simulink model "PMSM_Simulation"  (R2023a)
settings: Solver=ode23t  StartTime=0.0  StopTime=5  MaxStep=0.2  RelTol=1e-4  EnableMultiTasking=on
InitFcn:
  | p = 4;
  | Ld = 0.000425;
  | Lq = 0.00085;
  | psim = 0.119489;
  | Rs = 0.0485;
  | J = 0.00027;
  | Kpwm = 1;
  | Tsi = 0.0001;
  | h = 900;
  | 
  | L0 = (Ld+Lq)/2;
  | SMO_Kp = 100;
  | SMO_Coef =0.0001;
  | Ki_id = Ld*(h+1)/(4.5*Kpwm*(Tsi^2)*(h^2));
  | Kp_id = Ld*(h+1)/(4.5*Kpwm*Tsi*h);
  | 
  | wc =3000;
  | 
  | Ki_iq = Lq*(h+1)/(4.5*Kpwm*Tsi^2*h^2);
  | Kp_iq = Lq*(h+1)/(4.5*Kpwm*Tsi*h);
  | 
  | 
  | Kp_Spd = pi*J/(300*p*psim*Tsi)
  | Ki_Spd = pi*J/(6000*p*psim*Tsi^2)
  | 
  | DeadTime = 2e-6;
  | 
  | Udc = 650;
model workspace (MAT data in the model file):
  KfDeadCompen_CpPeriodTimesT_NULL = Simulink.Parameter
  KfDeadCompen_CpPeriodTimesT_NULL.Value = 0
  KfDeadCompen_CpPeriodTimesT_NULL.DataType = 'single'
  KfDeadCompen_CpPeriodTimesT_NULL.Complexity = 'real'
  KfDeadCompen_CpPeriodTimesT_NULL.Dimensions = [1 1]
  KfMDCC_InvParkCpPeriodTimesT_NULL = Simulink.Parameter
  KfMDCC_InvParkCpPeriodTimesT_NULL.Value = 0
  KfMDCC_InvParkCpPeriodTimesT_NULL.DataType = 'single'
  KfMDCC_InvParkCpPeriodTimesT_NULL.Complexity = 'real'
  KfMDCC_InvParkCpPeriodTimesT_NULL.Dimensions = [1 1]
values from neighbouring files (symbols this model uses):
  KfDeadCompen_SetDeltaTime_us = myPackage.Parameter    [DeadCompen.m]
  VbDeadComp_SwtUseIsttrDes_flg = myPackage.Parameter    [DeadCompen.m]
  VfDeadCompen_agIPredAdpr_C = myPackage.Parameter    [DeadCompen.m]
  VfDeadCompen_ISttrDdeThdSwt_A = myPackage.Parameter    [DeadCompen.m]
  VfDeadCompen_ISttrIgbtThdSwt_A = myPackage.Parameter    [DeadCompen.m]
  VfDeadCompen_rDdeISttrHi_R = myPackage.Parameter    [DeadCompen.m]
  VfDeadCompen_rDdeISttrLo_R = myPackage.Parameter    [DeadCompen.m]
  VfDeadCompen_rIgbtISttrHi_R = myPackage.Parameter    [DeadCompen.m]
  VfDeadCompen_rIgbtISttrLo_R = myPackage.Parameter    [DeadCompen.m]
  VfDeadCompen_uDdeISttrHi_V = myPackage.Parameter    [DeadCompen.m]
  VfDeadCompen_uDdeISttrLo_V = myPackage.Parameter    [DeadCompen.m]
  VfDeadCompen_uIgbtISttrHi_V = myPackage.Parameter    [DeadCompen.m]
  VfDeadCompen_uIgbtISttrLo_V = myPackage.Parameter    [DeadCompen.m]
undefined symbols (not defined in the file or in its folder): DiscIntNeverNeededParam, TableDeadTime_us, TableDeadTimeLookUpCur_A, VuDeadCompen_agIPredAdpr_C
libraries: simulink x23, mcbcontrolslib x11, mcbplantlib x1, spsCurrentMeasurementLib x1, spsDCVoltageSourceLib x1, spsMultimeterLib x1, spsPermanentMagnetSynchronousMachineLib x1, eePmsmCurrentController x1, spsThreePhaseVIMeasurementLib x1, spsUniversalBridgeLib x1, spspowerguiLib x1
(part 1 of 4)
settings Model: SimulationMode=accelerator  Creator=洲  LastModifiedBy=洲
settings SolverCC: AlgebraicLoopSolver=TrustRegion  MaxZcPerStep=1
settings DataIOCC: LimitDataPoints=on  MaxDataPoints=10000
settings OptimizationCC: ReuseModelBlockBuffer=off  LifeSpan=inf
settings DebuggingCC: AllowSymbolicDim=off  SFUnexpectedBacktrackingDiag=warning  SFNoUnconditionalDefaultTransitionDiag=warning  SFExecutionAtInitializationDiag=none  ArithmeticOperatorsInVariantConditions=warning
settings ModelReferenceCC: EnableRefExpFcnMdlSchedulingChecks=on
settings SFSimCC: SimUseLocalCustomCode=off  CustomCodeUndefinedFunction=UseInterfaceOnly
settings RTWCC: RTWUseLocalCustomCode=off  DLArmComputeVersion=19.05
settings CodeAppCC: StateflowObjectComments=on
settings GRTTargetCC: TargetLangStandard=C89/C90 (ANSI)
settings ConfigComp: CovMetricSettings=dw  CovSaveCumulativeToWorkspaceVar=on  CovSaveSingleToWorkspaceVar=on  CovExternalEMLEnable=off  CovSFcnEnable=off
settings SimscapeCC: SimscapeLogType=all  SimscapeLogDataHistory=10000

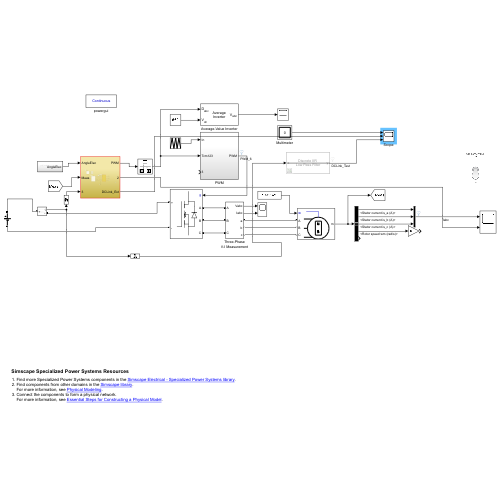
[thumbnail: Simulink's stored preview of the top-level diagram]
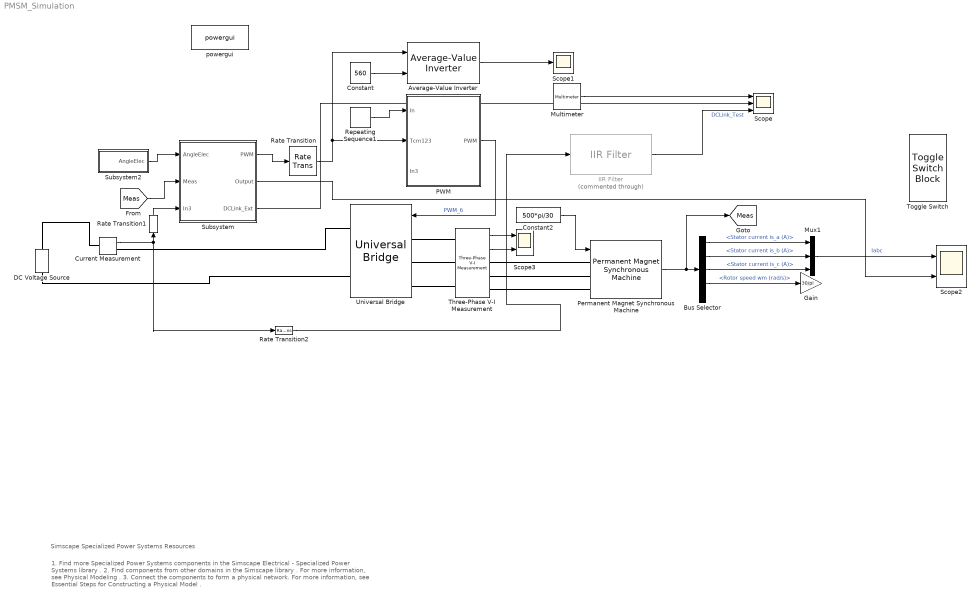
== system PMSM_Simulation ==
  note: 1. Find more Specialized Power Systems components in the Simscape Electrical - Specialized Power Systems library .
      | 2. Find components from other domains in the Simscape library .
      | For more information, see Physical Modeling .
      | 3. Connect the components to form a physical network.
      | For more information, see Essential Steps for Constructing a Physical Model .
  note: Simscape Specialized Power Systems Resources
  Average-Value Inverter : mcbplantlib/Average-Value Inverter
      settings: LibrarySourceBlock=mcblib/Electrical Systems/Inverters/Average-Value Inverter
  Bus Selector : BusSelector  OutputSignals=Stator current is_a (A),Stator current is_b (A),Stator current is_c (A),Rotor speed wm (rad/s),Electromagnetic torque Te (N*m)
  Constant : Constant  Value=560
  Constant2 : Constant  Value=500*pi/30
  Current Measurement : spsCurrentMeasurementLib/Current Measurement  PhasorSimulation=off  OutputType=Complex  PSBequivalent=0
  DC Voltage Source : spsDCVoltageSourceLib/DC Voltage Source  Amplitude=650  Measurements=None
  Gain : Gain  Gain=30/pi
  IIR Filter : mcbcontrolslib/IIR Filter  Commented=through  VariantControl=Low Pass Filter  VariantSelect=Low-pass  Filter_constant=0.0001  advancedSettings=off  Ts=50e-6  cutOff_freq=0.31834
      settings: LibrarySourceBlock=mcbhdllib/Signal Management/IIR Filter
  Multimeter : spsMultimeterLib/Multimeter  L=1  sel=1  yselected={}  Gain=0  OutputType=Complex  PlotAtSimulationStop=off  PhasorSimulation=off
  Mux1 : Mux  Inputs=3
  PWM : Subsystem
  Permanent Magnet Synchronous Machine : spsPermanentMagnetSynchronousMachineLib/Permanent Magnet Synchronous Machine  NbPhases=3  FluxDistribution=Sinusoidal  RotorType=Salient-pole  MechanicalLoad=Speed w  PresetModel=No  ShowDetailedParameters=on  MeasurementBus=off  Resistance=0.0485  Inductance=8.5e-3  dqInductances=[0.000425 0.00085]  La=0.000395  MachineConstant=Flux linkage established by magnets (V.s)  Flux=0.119489  VoltageCst=86.6916  TorqueCst=0.71693  Flat=120  Mechanical=[0.000621417 0.000303448 4]  PolePairs=4  InitialConditions=[0,0, 0,0]  InitialConditions5ph=[0 0 0 0 0 0]  RefAngle=Aligned with phase A axis (original Park)  IterativeDiscreteModel=Trapezoidal non iterative  TsBlock=-1  TsPowergui=0
  Rate Transition : RateTransition
  Rate Transition1 : RateTransition
  Rate Transition2 : RateTransition  OutPortSampleTime=0.0001
  Repeating Sequence1 : simulink/Sources/Repeating Sequence  rep_seq_t=[0 0.00005 0.0001]  rep_seq_y=[0 1 0]
  Scope : Scope  NumInputPorts=3
  Scope1 : Scope
  Scope2 : Scope  NumInputPorts=2
  Scope3 : Scope  NumInputPorts=2
  Subsystem : Subsystem  SystemSampleTime=0.0001
  Subsystem2 : Subsystem
  Three-Phase V-I Measurement : spsThreePhaseVIMeasurementLib/Three-Phase V-I Measurement  VoltageMeasurement=phase-to-phase  SetLabelV=off  LabelV=Vabc  Vpu=off  VpuLL=off  CurrentMeasurement=yes  SetLabelI=off  LabelI=Iabc  Ipu=off  Pbase=100e6  Vbase=500e3  OutputType=Complex  PhasorSimulation=off  PSBequivalent=0
  Toggle Switch : ToggleSwitchBlock
      settings: Values={{'Off', 'On'}, [0 1]}
  Universal Bridge : spsUniversalBridgeLib/Universal Bridge  Arms=3  SnubberResistance=1e5  SnubberCapacitance=inf  Device=MOSFET / Diodes  Ron=1e-3  Lon=0  ForwardVoltages="[  0  0  ]"  ForwardVoltage=0  GTOparameters=[ 10e-6 , 20e-6 ]  IGBTparameters=[ 1e-6 , 2e-6 ]  Measurements=None  Measurements_2=None  converterType=Rectifier
  powergui : spspowerguiLib/powergui  Priority=1  SimulationMode=Continuous  SampleTime=50e-6  frequency=60  Iterations=50  frequencyindice=0  Pbase=100e6  ErrMax=1e-4  UnitsV=kV  UnitsW=MW  buscounter=0  FunctionMessages=off  echomessages=off  EnableUseOfTLC=off  CurrentSourceSwitches=off  DisableSnubberDevices=off  DisableRonSwitches=off  DisableVfSwitches=off  DisplayEquations=off  AutomaticDiscreteSolvers=off  SolverType=Tustin/Backward Euler (TBE)  Interpol=off  ExternalGateDelay=off  methode=off  Ts=100  x0status=blocks  SPID=on  SwTol=0  HookPort=off  NonlinearTolerance=0  nMaxIteration=15  ContinueOnMaxIteration=off  RestoreLinks=warning  ResistiveCurrentMeasurement=off  Frange=[0:2:500]  Ylog=off  Xlog=on  ShowGrid=off  save=off  variable=ZData  structure=0  ZoomFFT=off  StartTime=0.0  cycles=1  DisplayStyle=1  fundamental=60  FreqAxis=off  MaxFrequency=1000  frequencyindicesteady=1  RmsSteady=1  display=off
  tag scope: Meas=global
  wires:
  Multimeter/1 -> Scope/1
  PWM/1(PWM) -> Universal Bridge/1  "PWM_6"
  Mux1/1 -> Scope2/1  "Iabc"
  Repeating Sequence1/1 -> PWM/1(In)
  Rate Transition/1 -> PWM/2(Tcm123), Average-Value Inverter/1
  Bus Selector/3 -> Mux1/3  "<Stator current is_c (A)>"
  Bus Selector/1 -> Mux1/1  "<Stator current is_a (A)>"
  [Meas] -> Subsystem/2(Meas)
  Bus Selector/2 -> Mux1/2  "<Stator current is_b (A)>"
  Permanent Magnet Synchronous Machine/1 -> [Meas], Bus Selector/1
  Subsystem/1(PWM) -> Rate Transition/1
  Subsystem2/1(AngleElec) -> Subsystem/1(AngleElec)
  Constant/1 -> Average-Value Inverter/2
  Average-Value Inverter/1 -> Scope1/1
  Bus Selector/4 -> Gain/1  "<Rotor speed wm (rad/s)>"
  Three-Phase V-I Measurement/1 -> Scope3/1
  Three-Phase V-I Measurement/2 -> Scope3/2
  Subsystem/2(Output) -> Scope2/2
  Constant2/1 -> Permanent Magnet Synchronous Machine/1
  Current Measurement/1 -> Rate Transition2/1, Rate Transition1/1
  Rate Transition1/1 -> Subsystem/3(In3)
  IIR Filter/1 -> Scope/3  "DCLink_Test"
  Subsystem/3(DCLink_Ext) -> Scope/2
  Rate Transition2/1 -> IIR Filter/1
  connections:
  Universal Bridge/RConn2 -- DC Voltage Source/LConn1
  DC Voltage Source/RConn1 -- Current Measurement/LConn1
  Three-Phase V-I Measurement/LConn2 -- Universal Bridge/LConn2
  Three-Phase V-I Measurement/LConn1 -- Universal Bridge/LConn1
  Three-Phase V-I Measurement/LConn3 -- Universal Bridge/LConn3
  Three-Phase V-I Measurement/RConn1 -- Permanent Magnet Synchronous Machine/LConn1
  Three-Phase V-I Measurement/RConn2 -- Permanent Magnet Synchronous Machine/LConn2
  Three-Phase V-I Measurement/RConn3 -- Permanent Magnet Synchronous Machine/LConn3
  Current Measurement/RConn1 -- Universal Bridge/RConn1

== system PMSM_Simulation/PWM ==
  In : Inport
  Tcm123 : Inport  Port=2
  In3 : Inport  Port=3
  Add : Sum  Inputs=+-
  Add1 : Sum  Inputs=+-
  Add2 : Sum  Inputs=+-
  Demux : Demux  Outputs=3
  Mux : Mux  Inputs=6
  Relay : Relay  OffSwitchValue=-eps
  Relay1 : Relay  OffSwitchValue=-eps
  Relay2 : Relay  OffSwitchValue=-eps
  Subsystem : Subsystem
  Subsystem1 : Subsystem
  Subsystem2 : Subsystem
  PWM : Outport
  wires:
  Demux/3 -> Add2/2
  Demux/2 -> Add1/2
  Demux/1 -> Add/2
  Add1/1 -> Relay1/1
  Add2/1 -> Relay2/1
  Add/1 -> Relay/1
  In/1 -> Add2/1, Add1/1, Add/1
  Tcm123/1 -> Demux/1
  Relay2/1 -> Subsystem2/1(PWM)
  Mux/1 -> PWM/1
  Relay/1 -> Subsystem/1(PWM)
  Subsystem/1(PWM_L) -> Mux/1
  Subsystem/2(PWM_H) -> Mux/2
  Relay1/1 -> Subsystem1/1(PWM)
  Subsystem1/1(PWM_L) -> Mux/3
  Subsystem1/2(PWM_H) -> Mux/4
  Subsystem2/2(PWM_H) -> Mux/6
  Subsystem2/1(PWM_L) -> Mux/5

== system PMSM_Simulation/Subsystem ==
  AngleElec : Inport
  Meas : Inport  Port=2
  In3 : Inport  Port=3
  Constant : Constant  Value=-50
  Constant1 : Constant  Value=100
  Function-Call Clock_50us : simulink/Ports & Subsystems/Function-Call Generator  sample_time=5e-5  numberOfIterations=1  DisallowWideOutput=off
  Function-Call Subsystem : Subsystem  TreatAsAtomicUnit=on
  Mux : Mux  Inputs=2
  Subsystem : Subsystem
  Task Scheduler : Stateflow chart  TreatAsAtomicUnit=on
  PWM : Outport
  Output : Outport  Port=2
  DCLink_Ext : Outport  Port=3
  wires:
  Task Scheduler/2(Task_100us_2()) -> [Task100us_2]
  Task Scheduler/3(Task_1ms_1()) -> [Task1ms_1]
  Function-Call Clock_50us/1 -> Task Scheduler/Trigger
  Task Scheduler/1(Task_100us_1()) -> [Task100us_1]
  [Task100us_1] -> Function-Call Subsystem/Trigger
  Meas/1 -> Function-Call Subsystem/1(Meas)
  Subsystem/1(PWM) -> PWM/1
  [Task100us_2] -> Subsystem/Trigger
  Function-Call Subsystem/3(Vdc) -> Subsystem/4(Vdc)
  Function-Call Subsystem/2(wElectrical) -> Subsystem/3(wElectrical)
  Function-Call Subsystem/1(iabc) -> Subsystem/2(Abc)
  Constant1/1 -> Mux/2
  Constant/1 -> Mux/1
  Mux/1 -> Subsystem/1(IdqRef)
  Function-Call Subsystem/4(theta) -> Subsystem/5(Theta)
  Subsystem/2(Output) -> Output/1
  In3/1 -> Subsystem/6(In6)
  Subsystem/3(DCLink_Ext) -> DCLink_Ext/1

== system PMSM_Simulation/Subsystem2 ==
  Add : Sum
  Constant3 : Constant  Value=5000
  Constant4 : Constant  Value=2*pi
  Delay : Delay  DelayLength=1
  Gain1 : Gain  Gain=pi/30
  Gain2 : Gain  Gain=0.0001
  Mod : Math  Operator=mod
  AngleElec : Outport
  wires:
  Add/1 -> Mod/1
  Gain2/1 -> Add/1
  Constant3/1 -> Gain1/1
  Mod/1 -> Delay/1, AngleElec/1
  Constant4/1 -> Mod/2
  Gain1/1 -> Gain2/1
  Delay/1 -> Add/2

== system PMSM_Simulation/PWM/Subsystem ==
  PWM : Inport
  Abs : Abs  SaturateOnIntegerOverflow=off
  Add3 : Sum  Inputs=+-
  Data Type Conversion : DataTypeConversion  OutDataTypeStr=double  SaturateOnIntegerOverflow=off  RndMeth=Floor
  Data Type Conversion3 : DataTypeConversion  OutDataTypeStr=double  SaturateOnIntegerOverflow=off  RndMeth=Floor
  Logical Operator : Logic  Operator=NOT  AllPortsSameDT=off  OutDataTypeStr=boolean
  Product : Product
  Product1 : Product
  Transport Delay1 : TransportDelay  DelayTime=DeadTime  BufferSize=1000
  PWM_L : Outport
  PWM_H : Outport  Port=2
  wires:
  Product/1 -> PWM_L/1
  Add3/1 -> Abs/1
  PWM/1 -> Logical Operator/1, Data Type Conversion3/1
  Transport Delay1/1 -> Add3/2, Product1/2
  Logical Operator/1 -> Data Type Conversion/1
  Data Type Conversion/1 -> Product/1, Add3/1
  Data Type Conversion3/1 -> Transport Delay1/1
  Product1/1 -> PWM_H/1
  Abs/1 -> Product1/1, Product/2

== system PMSM_Simulation/PWM/Subsystem1 ==
  PWM : Inport
  Abs : Abs  SaturateOnIntegerOverflow=off
  Add3 : Sum  Inputs=+-
  Data Type Conversion : DataTypeConversion  OutDataTypeStr=double  SaturateOnIntegerOverflow=off  RndMeth=Floor
  Data Type Conversion3 : DataTypeConversion  OutDataTypeStr=double  SaturateOnIntegerOverflow=off  RndMeth=Floor
  Logical Operator : Logic  Operator=NOT  AllPortsSameDT=off  OutDataTypeStr=boolean
  Product : Product
  Product1 : Product
  Transport Delay1 : TransportDelay  DelayTime=DeadTime  BufferSize=1000
  PWM_L : Outport
  PWM_H : Outport  Port=2
  wires:
  Product/1 -> PWM_L/1
  Add3/1 -> Abs/1
  PWM/1 -> Logical Operator/1, Data Type Conversion3/1
  Transport Delay1/1 -> Add3/2, Product1/2
  Logical Operator/1 -> Data Type Conversion/1
  Data Type Conversion/1 -> Product/1, Add3/1
  Data Type Conversion3/1 -> Transport Delay1/1
  Product1/1 -> PWM_H/1
  Abs/1 -> Product1/1, Product/2

== system PMSM_Simulation/PWM/Subsystem2 ==
  PWM : Inport
  Abs : Abs  SaturateOnIntegerOverflow=off
  Add3 : Sum  Inputs=+-
  Data Type Conversion : DataTypeConversion  OutDataTypeStr=double  SaturateOnIntegerOverflow=off  RndMeth=Floor
  Data Type Conversion3 : DataTypeConversion  OutDataTypeStr=double  SaturateOnIntegerOverflow=off  RndMeth=Floor
  Logical Operator : Logic  Operator=NOT  AllPortsSameDT=off  OutDataTypeStr=boolean
  Product : Product
  Product1 : Product
  Transport Delay1 : TransportDelay  DelayTime=DeadTime  BufferSize=1000
  PWM_L : Outport
  PWM_H : Outport  Port=2
  wires:
  Product/1 -> PWM_L/1
  Add3/1 -> Abs/1
  PWM/1 -> Logical Operator/1, Data Type Conversion3/1
  Transport Delay1/1 -> Add3/2, Product1/2
  Logical Operator/1 -> Data Type Conversion/1
  Data Type Conversion/1 -> Product/1, Add3/1
  Data Type Conversion3/1 -> Transport Delay1/1
  Product1/1 -> PWM_H/1
  Abs/1 -> Product1/1, Product/2

== system PMSM_Simulation/Subsystem/Function-Call Subsystem ==
  Meas : Inport
  function : TriggerPort  TriggerType=function-call  VariantControl=(inherit)
  Add : Sum
  Bus Selector : BusSelector  OutputSignals=Stator current is_a (A),Stator current is_b (A),Stator current is_c (A),Rotor angle thetam (rad),Rotor speed wm (rad/s)
  Constant : Constant  Value=2*pi  SampleTime=-1
  Constant1 : Constant  Value=650
  Constant2 : Constant  Value=500*pi/30
  Constant3 : Constant  Value=2*pi
  Delay : Delay  DelayLength=1
  Gain : Gain  Gain=0.0001
  Math Function : Math  Operator=mod  SignedPower=on
  Mod : Math  Operator=mod
  Mux : Mux  Inputs=3
  pole pairs1 : Gain  Gain=p
  pole pairs2 : Gain  Gain=p
  iabc : Outport
  wElectrical : Outport  Port=2  VectorParamsAs1DForOutWhenUnconnected=off
  Vdc : Outport  Port=3  VectorParamsAs1DForOutWhenUnconnected=off
  theta : Outport  Port=4  VectorParamsAs1DForOutWhenUnconnected=off
  wires:
  Meas/1 -> Bus Selector/1
  Math Function/1 -> theta/1
  Constant/1 -> Math Function/2
  pole pairs1/1 -> Math Function/1
  pole pairs2/1 -> Add/1
  Bus Selector/4 -> pole pairs1/1  "<Rotor angle thetam (rad)>"
  Bus Selector/2 -> Mux/2  "<Stator current is_b (A)>"
  Bus Selector/1 -> Mux/1  "<Stator current is_a (A)>"
  Bus Selector/3 -> Mux/3  "<Stator current is_c (A)>"
  Mux/1 -> iabc/1
  Constant1/1 -> Vdc/1
  Constant2/1 -> Gain/1
  Gain/1 -> pole pairs2/1
  Add/1 -> Mod/1
  Delay/1 -> Add/2
  Constant3/1 -> Mod/2
  Mod/1 -> wElectrical/1, Delay/1

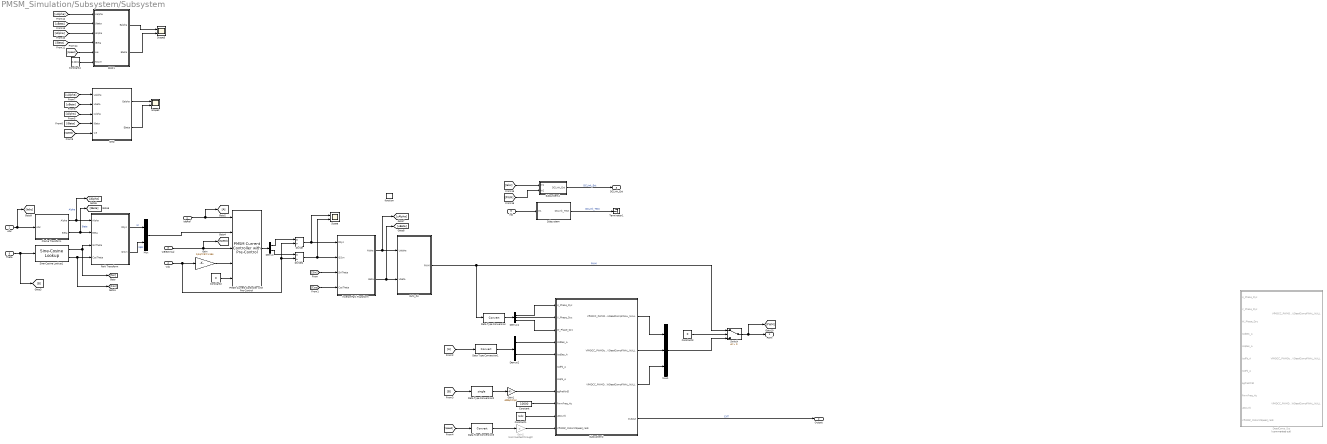
== system PMSM_Simulation/Subsystem/Subsystem ==
  IdqRef : Inport
  Abc : Inport  Port=2
  wElectrical : Inport  Port=3
  Vdc : Inport  Port=4  OutMin=100
  Theta : Inport  Port=5
  In6 : Inport  Port=6
  function : TriggerPort  TriggerType=function-call  VariantControl=(inherit)
  Clarke Transform : Subsystem  TreatAsAtomicUnit=on
      settings: RTWSystemCode=Nonreusable function
  Constant : Constant  Value=10000  OutDataTypeStr=single
  Constant1 : Constant  Value=Udc  OutDataTypeStr=single
  Constant2 : Constant  Value=0
  Constant3 : Constant  Value=0
  Constant4 : Constant  Value=0.0001
  Data Type Conversion : DataTypeConversion  SaturateOnIntegerOverflow=off  RndMeth=Floor
  Data Type Conversion1 : DataTypeConversion  SaturateOnIntegerOverflow=off  RndMeth=Floor
  Data Type Conversion2 : DataTypeConversion  OutDataTypeStr=single  SaturateOnIntegerOverflow=off  RndMeth=Floor
  Data Type Conversion3 : DataTypeConversion  SaturateOnIntegerOverflow=off  RndMeth=Floor
  DeadComp_Sys : Subsystem  Commented=on  TreatAsAtomicUnit=on
      settings: RTWSystemCode=Nonreusable function
  Demux : Demux  Outputs=2
  Demux1 : Demux  Outputs=3
  Demux2 : Demux  Outputs=2
  Divide : Product  Inputs=*/
  Divide1 : Product  Inputs=*/
  From2 : From
  Gain : Gain  Gain=1/sqrt(3)*1.154
  Gain1 : Gain  Gain=4095/(2*pi)
  Gain2 : Gain  Commented=through  Gain=p
  Goto2 : Goto
  Inverse Park Transform : Subsystem  TreatAsAtomicUnit=on
  Mux : Mux  Inputs=2
  Mux1 : Mux  Inputs=3
  PMSM Current Controller with Pre-Control : eePmsmCurrentController/PMSM Current Controller with Pre-Control  Kp_id=Kp_id  Ki_id=Ki_id  Kaw_id=1  Kp_iq=Kp_iq  Ki_iq=Ki_iq  Kaw_iq=1  Ts=-1  Tsd=Tsi  AxisPrio=D-axis  ActZC=on  ActFF=on  idVect=[-200, 0, 200]  iqVect=[-200, 0, 200]  LdMatrix=Ld * ones(3, 3)  LqMatrix=Lq * ones(3, 3)  psimMatrix=psim * ones(3, 3)
  Park Transform : Subsystem  TreatAsAtomicUnit=on
      settings: RTWSystemCode=Nonreusable function
  SMO : Subsystem
  SMO1 : Subsystem
  SVM_PU : Subsystem  TreatAsAtomicUnit=on  RTWFcnName=SVPWM_Calc
      settings: RTWSystemCode=Nonreusable function  RTWFcnNameOpts=User specified
  Scope : Scope  NumInputPorts=2
  Scope2 : Scope  NumInputPorts=2
  Scope3 : Scope  NumInputPorts=2
  Sine-Cosine Lookup1 : mcbcontrolslib/Sine-Cosine Lookup  AngleInput=Radians  N_points=4095
      settings: LibrarySourceBlock=mcblib/Controls/Math Transforms/Sine-Cosine Lookup
  Subsystem : Subsystem
  Subsystem2 : Subsystem
  Subsystem4 : Subsystem
  Switch : Switch  Criteria=u2 > Threshold  SaturateOnIntegerOverflow=off  InputSameDT=off
  Terminator1 : Terminator
  PWM : Outport
  Output : Outport  Port=2
  DCLink_Ext : Outport  Port=3
  wires:
  Inverse Park Transform/2(Beta) -> [uBeta], SVM_PU/2(Ubeta)
  Inverse Park Transform/1(Alpha) -> [uAlpha], SVM_PU/1(Ualpha)
  SVM_PU/1(PWM) -> Data Type Conversion/1, Switch/1  "PWM"
  wElectrical/1 -> [Speed], PMSM Current Controller with Pre-Control/3
  Sine-Cosine Lookup1/2 -> [Cos], Park Transform/4(CosTheta)
  Park Transform/2(QSyn) -> Mux/2  "IqBk"
  Mux/1 -> PMSM Current Controller with Pre-Control/2
  Gain/1 -> PMSM Current Controller with Pre-Control/4
  Vdc/1 -> Divide/2, Divide1/2, Gain/1
  Sine-Cosine Lookup1/1 -> [Sin], Park Transform/3(SinTheta)
  IdqRef/1 -> Goto2/1, PMSM Current Controller with Pre-Control/1
  Constant2/1 -> PMSM Current Controller with Pre-Control/5
  Theta/1 -> [B], Sine-Cosine Lookup1/1
  Clarke Transform/1(Alpha) -> [iAlpha], Park Transform/1(Alpha)  "Alpha"
  Clarke Transform/2(Beta) -> [iBeta], Park Transform/2(Beta)  "Beta"
  Abc/1 -> [Iabc], Clarke Transform/1(Abc)
  Park Transform/1(DSyn) -> Mux/1  "id"
  [Sin] -> Inverse Park Transform/3(SinTheta)
  [Cos] -> Inverse Park Transform/4(CosTheta)
  PMSM Current Controller with Pre-Control/1 -> Demux/1
  Demux/1 -> Divide/1
  Demux/2 -> Divide1/1
  Demux1/2 -> Subsystem2/2(V_Phase_Dyc)
  Demux1/1 -> Subsystem2/1(U_Phase_Dyc)
  Demux1/3 -> Subsystem2/3(W_Phase_Dyc)
  Demux2/1 -> Subsystem2/4(IsdDes_A)
  Demux2/2 -> Subsystem2/5(IsqDes_A)
  From2/1 -> Data Type Conversion1/1
  [B] -> Data Type Conversion2/1
  Gain1/1 -> Subsystem2/8(agPreRtrEl)
  Constant/1 -> Subsystem2/9(PwmFreq_Hz)
  Constant1/1 -> Subsystem2/10(uDcLink)
  [Speed] -> Data Type Conversion3/1
  Gain2/1 -> Subsystem2/11(VfMDSP_MotorMSpeed_rads)
  Subsystem2/2(VfMDCC_PWMDutyVDeadCompFINAL_NULL) -> Mux1/2
  Subsystem2/1(VfMDCC_PWMDutyUDeadCompFINAL_NULL) -> Mux1/1
  Subsystem2/3(VfMDCC_PWMDutyWDeadCompFINAL_NULL) -> Mux1/3
  Mux1/1 -> Switch/3
  Switch/1 -> [PWM], PWM/1
  Constant3/1 -> Switch/2
  Data Type Conversion/1 -> Demux1/1
  Data Type Conversion1/1 -> Demux2/1
  Data Type Conversion2/1 -> Gain1/1
  Data Type Conversion3/1 -> Gain2/1
  Subsystem2/4(Output) -> Output/1  "CNT"
  Divide/1 -> Inverse Park Transform/1(DSyn), Scope/1
  Divide1/1 -> Inverse Park Transform/2(QSyn), Scope/2
  [iBeta] -> SMO/4(iBeta)
  [iAlpha] -> SMO/3(iAlpha)
  [uAlpha] -> SMO/1(Ualpha)
  [uBeta] -> SMO/2(Ubeta)
  [Speed] -> SMO/5(we)
  SMO/1(Ealpha) -> Scope2/1
  SMO/2(Ebeta) -> Scope2/2
  [uAlpha] -> SMO1/1(Ualpha)
  [uBeta] -> SMO1/2(Ubeta)
  [iAlpha] -> SMO1/3(iAlpha)
  [iBeta] -> SMO1/4(iBeta)
  Constant4/1 -> SMO1/6(Tpwm)
  SMO1/1(Ealpha) -> Scope3/1
  SMO1/2(Ebeta) -> Scope3/2
  [Speed] -> SMO1/5(we)
  [Iabc] -> Subsystem4/1(In1)
  [PWM] -> Subsystem4/2(In2)
  Subsystem4/1(DCLink_Ext) -> DCLink_Ext/1  "DCLink_Ext"
  In6/1 -> Subsystem/1(In1)
  Subsystem/1(DCLink_Test) -> Terminator1/1  "DCLink_Test"

== system PMSM_Simulation/Subsystem/Subsystem/Clarke Transform ==
  Abc : Inport
  Add : Sum  Inputs=+++
  Add1 : Sum
  Demux : Demux  Outputs=3
  Gain : Gain  Gain=2/3
  Gain1 : Gain  Gain=-1/3
  Gain2 : Gain  Gain=sqrt(3)/3
  Gain3 : Gain  Gain=-sqrt(3)/3
  Gain4 : Gain  Gain=-1/3
  Alpha : Outport  VectorParamsAs1DForOutWhenUnconnected=off
  Beta : Outport  Port=2  VectorParamsAs1DForOutWhenUnconnected=off
  wires:
  Gain3/1 -> Add1/2
  Demux/3 -> Gain3/1, Gain4/1
  Add1/1 -> Beta/1
  Demux/2 -> Gain2/1, Gain1/1
  Add/1 -> Alpha/1
  Gain2/1 -> Add1/1
  Gain1/1 -> Add/2
  Demux/1 -> Gain/1
  Gain/1 -> Add/1
  Abc/1 -> Demux/1
  Gain4/1 -> Add/3

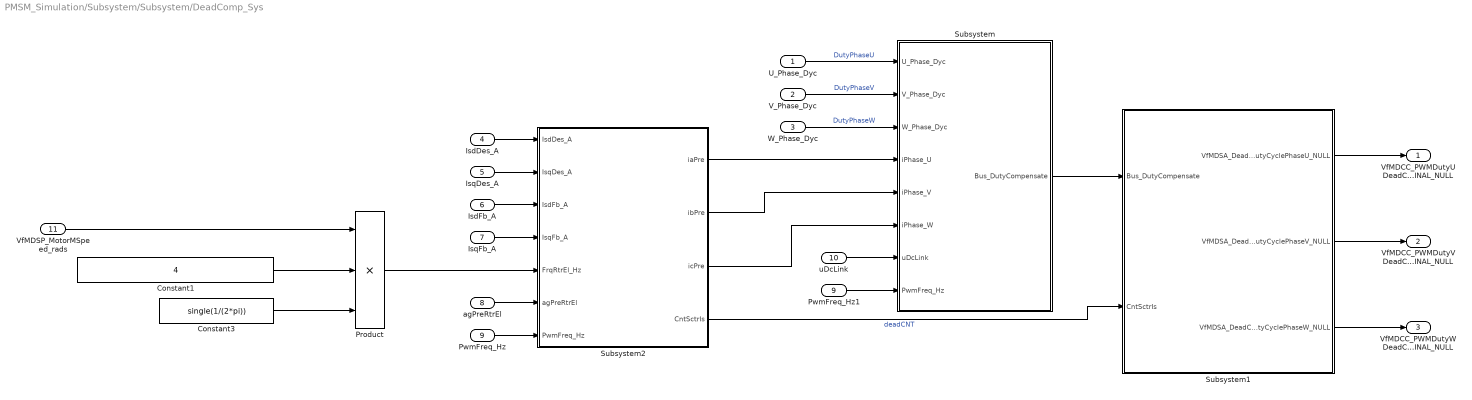
== system PMSM_Simulation/Subsystem/Subsystem/DeadComp_Sys ==
  U_Phase_Dyc : Inport
  V_Phase_Dyc : Inport  Port=2
  W_Phase_Dyc : Inport  Port=3
  IsdDes_A : Inport  Port=4
  IsqDes_A : Inport  Port=5
  IsdFb_A : Inport  Port=6
  IsqFb_A : Inport  Port=7
  agPreRtrEl : Inport  Port=8
  PwmFreq_Hz : Inport  Port=9
  uDcLink : Inport  Port=10
  VfMDSP_MotorMSpeed_rads : Inport  Port=11
  Constant1 : Constant  Value=4
  Constant3 : Constant  Value=single(1/(2*pi))
  Product : Product  Inputs=3
  PwmFreq_Hz1 : InportShadow  Port=9
  Subsystem : Subsystem
  Subsystem1 : Subsystem
  Subsystem2 : Subsystem
  VfMDCC_PWMDutyUDeadCompFINAL_NULL : Outport
  VfMDCC_PWMDutyVDeadCompFINAL_NULL : Outport  Port=2
  VfMDCC_PWMDutyWDeadCompFINAL_NULL : Outport  Port=3
  wires:
  IsdFb_A/1 -> Subsystem2/3(IsdFb_A)
  IsqFb_A/1 -> Subsystem2/4(IsqFb_A)
  Product/1 -> Subsystem2/5(FrqRtrEl_Hz)
  agPreRtrEl/1 -> Subsystem2/6(agPreRtrEl)
  Subsystem2/4(CntSctrIs) -> Subsystem1/2(CntSctrIs)  "deadCNT"
  IsqDes_A/1 -> Subsystem2/2(IsqDes_A)
  IsdDes_A/1 -> Subsystem2/1(IsdDes_A)
  U_Phase_Dyc/1 -> Subsystem/1(U_Phase_Dyc)  "DutyPhaseU"
  Subsystem2/1(iaPre) -> Subsystem/4(iPhase_U)
  V_Phase_Dyc/1 -> Subsystem/2(V_Phase_Dyc)  "DutyPhaseV"
  Subsystem2/2(ibPre) -> Subsystem/5(iPhase_V)
  Subsystem2/3(icPre) -> Subsystem/6(iPhase_W)
  W_Phase_Dyc/1 -> Subsystem/3(W_Phase_Dyc)  "DutyPhaseW"
  PwmFreq_Hz/1 -> Subsystem2/7(PwmFreq_Hz)
  uDcLink/1 -> Subsystem/7(uDcLink)
  Constant1/1 -> Product/2
  VfMDSP_MotorMSpeed_rads/1 -> Product/1
  Constant3/1 -> Product/3
  Subsystem1/1(VfMDSA_DeadCompPwmDutyCyclePhaseU_NULL) -> VfMDCC_PWMDutyUDeadCompFINAL_NULL/1
  Subsystem1/2(VfMDSA_DeadCompPwmDutyCyclePhaseV_NULL) -> VfMDCC_PWMDutyVDeadCompFINAL_NULL/1
  Subsystem1/3(VfMDSA_DeadCompPwmDutyCyclePhaseW_NULL) -> VfMDCC_PWMDutyWDeadCompFINAL_NULL/1
  PwmFreq_Hz1/1 -> Subsystem/8(PwmFreq_Hz)
  Subsystem/1(Bus_DutyCompensate) -> Subsystem1/1(Bus_DutyCompensate)

== system PMSM_Simulation/Subsystem/Subsystem/Inverse Park Transform ==
  DSyn : Inport
  QSyn : Inport  Port=2
  SinTheta : Inport  Port=3
  CosTheta : Inport  Port=4
  Add : Sum
  Add1 : Sum  Inputs=+-
  CosTheta1 : InportShadow  Port=4
  DSyn1 : InportShadow
  Product{,1..3} (4 alike) : Product  RndMeth=Zero
  QSyn1 : InportShadow  Port=2
  SinTheta1 : InportShadow  Port=3
  Alpha : Outport  VectorParamsAs1DForOutWhenUnconnected=off
  Beta : Outport  Port=2  VectorParamsAs1DForOutWhenUnconnected=off
  wires:
  SinTheta/1 -> Product3/2
  DSyn/1 -> Product2/1
  QSyn1/1 -> Product1/1
  DSyn1/1 -> Product/1
  SinTheta1/1 -> Product/2
  CosTheta1/1 -> Product1/2
  Product1/1 -> Add/2
  Product2/1 -> Add1/1
  QSyn/1 -> Product3/1
  Add/1 -> Beta/1
  Product/1 -> Add/1
  Product3/1 -> Add1/2
  Add1/1 -> Alpha/1
  CosTheta/1 -> Product2/2

== system PMSM_Simulation/Subsystem/Subsystem/Park Transform ==
  Alpha : Inport
  Beta : Inport  Port=2
  SinTheta : Inport  Port=3
  CosTheta : Inport  Port=4
  Add : Sum  Inputs=-+
  Add1 : Sum
  Alpha1 : InportShadow
  Beta1 : InportShadow  Port=2
  CosTheta1 : InportShadow  Port=4
  Product{,1..3} (4 alike) : Product  RndMeth=Zero
  SineTheta1 : InportShadow  Port=3
  DSyn : Outport  VectorParamsAs1DForOutWhenUnconnected=off
  QSyn : Outport  Port=2  VectorParamsAs1DForOutWhenUnconnected=off
  wires:
  Product1/1 -> Add/2
  Product/1 -> Add/1
  Product3/1 -> Add1/2
  Add1/1 -> DSyn/1
  Beta1/1 -> Product1/1
  Alpha1/1 -> Product/1
  SineTheta1/1 -> Product/2
  Product2/1 -> Add1/1
  Beta/1 -> Product3/1
  CosTheta/1 -> Product2/2
  Add/1 -> QSyn/1
  Alpha/1 -> Product2/1
  CosTheta1/1 -> Product1/2
  SinTheta/1 -> Product3/2

== system PMSM_Simulation/Subsystem/Subsystem/SMO ==
  Ualpha : Inport
  Ubeta : Inport  Port=2
  iAlpha : Inport  Port=3
  iBeta : Inport  Port=4
  we : Inport  Port=5
  Subsystem : Subsystem
  Subsystem1 : Subsystem
  Ealpha : Outport
  Ebeta : Outport  Port=2
  wires:
  iAlpha/1 -> Subsystem/2(iAlpha)
  Subsystem1/1(iBeta’) -> Subsystem/4(iBeta‘)  "iBeta’"
  Ualpha/1 -> Subsystem/1(Ualpha)
  Subsystem/1(Ealpha) -> Ealpha/1  "Ealpha"
  we/1 -> Subsystem1/2(we), Subsystem/3(we)
  Subsystem/2(Ialpha’) -> Subsystem1/1(iAlpha')  "Ialpha’"
  iBeta/1 -> Subsystem1/4(iBeta)
  Ubeta/1 -> Subsystem1/3(Ubeta)
  Subsystem1/2(Ebeta) -> Ebeta/1  "Ebeta"

== system PMSM_Simulation/Subsystem/Subsystem/SMO1 ==
  Ualpha : Inport
  Ubeta : Inport  Port=2
  iAlpha : Inport  Port=3
  iBeta : Inport  Port=4
  we : Inport  Port=5
  Tpwm : Inport  Port=6
  Ealpha_calc : Subsystem
  Ebeta_Calc : Subsystem
  Scope : Scope  NumInputPorts=2
  Ealpha : Outport
  Ebeta : Outport  Port=2
  wires:
  we/1 -> Ebeta_Calc/2(we), Ealpha_calc/3(we)
  Ualpha/1 -> Ealpha_calc/1(Ualpha)
  Ubeta/1 -> Ebeta_Calc/4(Ubeta)
  Tpwm/1 -> Ebeta_Calc/3(Tpwm), Ealpha_calc/4(Tpwm)
  iAlpha/1 -> Ealpha_calc/2(iAlpha)
  Ealpha_calc/2(ialpha) -> Scope/1, Ebeta_Calc/1(ialpha')  "alpha_i"
  Ealpha_calc/1(Ealpha) -> Ealpha/1
  Ebeta_Calc/1(ibeta) -> Ealpha_calc/5(iBeta'), Scope/2  "beta_i"
  iBeta/1 -> Ebeta_Calc/5(iBeta)
  Ebeta_Calc/2(Ebeta) -> Ebeta/1

== system PMSM_Simulation/Subsystem/Subsystem/SVM_PU ==
  Ualpha : Inport
  Ubeta : Inport  Port=2
  Add : Sum  Inputs=+-
  Add1 : Sum  Inputs=+-
  Add2 : Sum  Inputs=+-
  Bus Selector : BusSelector  OutputSignals=Tcm1,Tcm2,Tcm3
  Constant : Constant  OutDataTypeStr=single
  Gain : Gain  Gain=2
  Gain1 : Gain  Gain=2
  Gain2 : Gain  Gain=2
  Mux : Mux  Inputs=3
  N_Sector_calc : Subsystem
  Subsystem : Subsystem
  Subsystem1 : Subsystem
  T1_T2_Calc : Subsystem
  Tcm_Calc : Subsystem
  PWM : Outport
  wires:
  Ualpha/1 -> Subsystem/1(Ualpha), N_Sector_calc/1(Ualpha)
  Ubeta/1 -> Subsystem/2(Ubeta), N_Sector_calc/2(Ubeta)
  N_Sector_calc/1(N_Sector) -> Tcm_Calc/1(N_Sector), T1_T2_Calc/1(N_Sector)
  Subsystem/1(X) -> T1_T2_Calc/2(X)
  Subsystem/2(Y) -> T1_T2_Calc/3(Y)
  Subsystem/3(Z) -> T1_T2_Calc/4(Z)
  Subsystem1/1(Ta) -> Tcm_Calc/2(Ta)
  Subsystem1/2(Tb) -> Tcm_Calc/3(Tb)
  Subsystem1/3(Tc) -> Tcm_Calc/4(Tc)
  Tcm_Calc/1(Bus_CMP) -> Bus Selector/1
  T1_T2_Calc/1(T1) -> Subsystem1/1(T1)
  T1_T2_Calc/2(T2) -> Subsystem1/2(T2)
  Bus Selector/1 -> Gain/1  "<Tcm1>"
  Bus Selector/2 -> Gain1/1  "<Tcm2>"
  Bus Selector/3 -> Gain2/1  "<Tcm3>"
  Constant/1 -> Add2/1, Add1/1, Add/1
  Gain/1 -> Add/2
  Gain1/1 -> Add1/2
  Gain2/1 -> Add2/2
  Add/1 -> Mux/1
  Add1/1 -> Mux/2
  Add2/1 -> Mux/3
  Mux/1 -> PWM/1

== system PMSM_Simulation/Subsystem/Subsystem/Subsystem ==
  In1 : Inport
  IIR Filter : mcbcontrolslib/IIR Filter  Commented=through  VariantControl=Low Pass Filter  VariantSelect=Low-pass  Filter_constant=0.0001  advancedSettings=off  Ts=50e-6  cutOff_freq=0.31834
      settings: LibrarySourceBlock=mcbhdllib/Signal Management/IIR Filter
  DCLink_Test : Outport
  wires:
  IIR Filter/1 -> DCLink_Test/1  "DCLink_Test"
  In1/1 -> IIR Filter/1

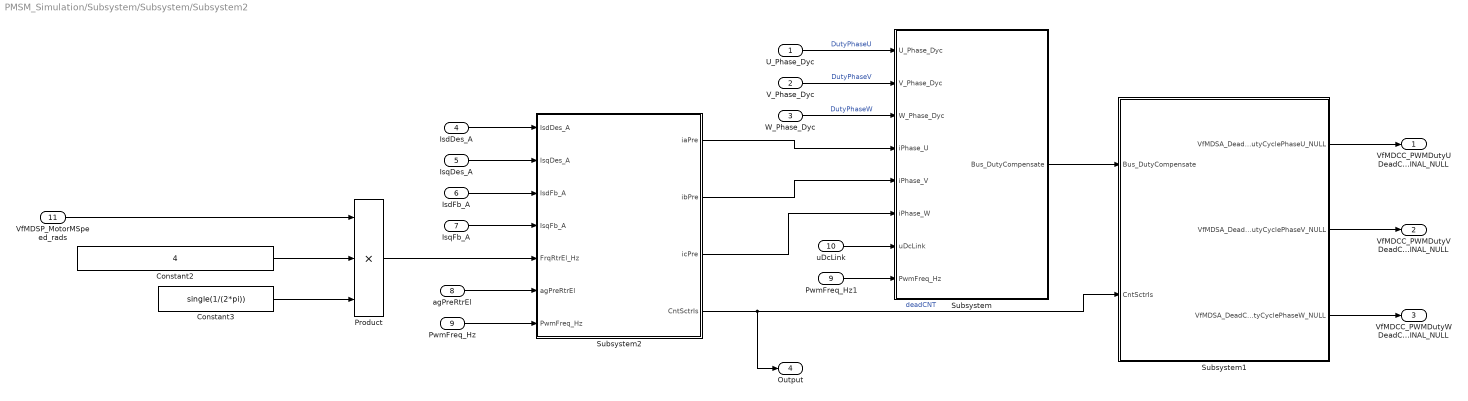
== system PMSM_Simulation/Subsystem/Subsystem/Subsystem2 ==
  U_Phase_Dyc : Inport
  V_Phase_Dyc : Inport  Port=2
  W_Phase_Dyc : Inport  Port=3
  IsdDes_A : Inport  Port=4
  IsqDes_A : Inport  Port=5
  IsdFb_A : Inport  Port=6
  IsqFb_A : Inport  Port=7
  agPreRtrEl : Inport  Port=8
  PwmFreq_Hz : Inport  Port=9
  uDcLink : Inport  Port=10
  VfMDSP_MotorMSpeed_rads : Inport  Port=11
  Constant2 : Constant  Value=4  OutDataTypeStr=single
  Constant3 : Constant  Value=single(1/(2*pi))
  Product : Product  Inputs=3
  PwmFreq_Hz1 : InportShadow  Port=9
  Subsystem : Subsystem
  Subsystem1 : Subsystem
  Subsystem2 : Subsystem
  VfMDCC_PWMDutyUDeadCompFINAL_NULL : Outport
  VfMDCC_PWMDutyVDeadCompFINAL_NULL : Outport  Port=2
  VfMDCC_PWMDutyWDeadCompFINAL_NULL : Outport  Port=3
  Output : Outport  Port=4
  wires:
  IsdFb_A/1 -> Subsystem2/3(IsdFb_A)
  IsqFb_A/1 -> Subsystem2/4(IsqFb_A)
  Product/1 -> Subsystem2/5(FrqRtrEl_Hz)
  agPreRtrEl/1 -> Subsystem2/6(agPreRtrEl)
  Subsystem2/4(CntSctrIs) -> Output/1, Subsystem1/2(CntSctrIs)  "deadCNT"
  IsqDes_A/1 -> Subsystem2/2(IsqDes_A)
  IsdDes_A/1 -> Subsystem2/1(IsdDes_A)
  U_Phase_Dyc/1 -> Subsystem/1(U_Phase_Dyc)  "DutyPhaseU"
  Subsystem2/1(iaPre) -> Subsystem/4(iPhase_U)
  V_Phase_Dyc/1 -> Subsystem/2(V_Phase_Dyc)  "DutyPhaseV"
  Subsystem2/2(ibPre) -> Subsystem/5(iPhase_V)
  Subsystem2/3(icPre) -> Subsystem/6(iPhase_W)
  W_Phase_Dyc/1 -> Subsystem/3(W_Phase_Dyc)  "DutyPhaseW"
  PwmFreq_Hz/1 -> Subsystem2/7(PwmFreq_Hz)
  uDcLink/1 -> Subsystem/7(uDcLink)
  Constant2/1 -> Product/2
  VfMDSP_MotorMSpeed_rads/1 -> Product/1
  Constant3/1 -> Product/3
  Subsystem1/1(VfMDSA_DeadCompPwmDutyCyclePhaseU_NULL) -> VfMDCC_PWMDutyUDeadCompFINAL_NULL/1
  Subsystem1/2(VfMDSA_DeadCompPwmDutyCyclePhaseV_NULL) -> VfMDCC_PWMDutyVDeadCompFINAL_NULL/1
  Subsystem1/3(VfMDSA_DeadCompPwmDutyCyclePhaseW_NULL) -> VfMDCC_PWMDutyWDeadCompFINAL_NULL/1
  PwmFreq_Hz1/1 -> Subsystem/8(PwmFreq_Hz)
  Subsystem/1(Bus_DutyCompensate) -> Subsystem1/1(Bus_DutyCompensate)

== system PMSM_Simulation/Subsystem/Subsystem/Subsystem4 ==
  In1 : Inport
  In2 : Inport  Port=2
  Add : Sum  Inputs=+++
  Delay : Delay  DelayLength=1
  Delay1 : Delay  DelayLength=1
  Delay2 : Delay  DelayLength=1
  Demux : Demux  Outputs=3
  Demux1 : Demux  Outputs=3
  IIR Filter1 : mcbcontrolslib/IIR Filter  Commented=through  VariantControl=Low Pass Filter  VariantSelect=Low-pass  Filter_constant=0.0001  advancedSettings=off  Ts=50e-6  cutOff_freq=0.31834
      settings: LibrarySourceBlock=mcbhdllib/Signal Management/IIR Filter
  Subsystem1 : Subsystem
  Subsystem2 : Subsystem
  Subsystem3 : Subsystem
  DCLink_Ext : Outport
  wires:
  Demux1/2 -> Subsystem2/2(In2)
  Subsystem3/1(Out1) -> Add/3
  Demux/1 -> Delay/1
  Subsystem1/1(Out1) -> Add/1
  Delay/1 -> Subsystem1/1(In1)
  Subsystem2/1(Out1) -> Add/2
  Demux/2 -> Delay1/1
  Demux1/3 -> Subsystem3/2(In2)
  Delay2/1 -> Subsystem3/1(In1)
  Demux/3 -> Delay2/1
  Delay1/1 -> Subsystem2/1(In1)
  Add/1 -> IIR Filter1/1
  Demux1/1 -> Subsystem1/2(In2)
  In1/1 -> Demux1/1
  IIR Filter1/1 -> DCLink_Ext/1  "DCLink_Ext"
  In2/1 -> Demux/1

== system PMSM_Simulation/Subsystem/Subsystem/DeadComp_Sys/Subsystem ==
  U_Phase_Dyc : Inport
  V_Phase_Dyc : Inport  Port=2
  W_Phase_Dyc : Inport  Port=3
  iPhase_U : Inport  Port=4
  iPhase_V : Inport  Port=5
  iPhase_W : Inport  Port=6
  uDcLink : Inport  Port=7
  PwmFreq_Hz : Inport  Port=8
  Bus Creator : BusCreator  Inputs=4
  Bus Creator1 : BusCreator  Inputs=3
  DeadTimeDuty_Calc : Subsystem
  DeltaTimeOnOffDuty_Calc : Subsystem
  Tavon_Calc : Subsystem
  Bus_DutyCompensate : Outport
  wires:
  U_Phase_Dyc/1 -> Bus Creator1/1, Tavon_Calc/1(U_Phase_Dyc)  "DutyPhaseU"
  V_Phase_Dyc/1 -> Bus Creator1/2, Tavon_Calc/2(V_Phase_Dyc)  "DutyPhaseV"
  W_Phase_Dyc/1 -> Bus Creator1/3, Tavon_Calc/3(W_Phase_Dyc)  "DutyPhaseW"
  iPhase_U/1 -> DeltaTimeOnOffDuty_Calc/1(iPhase_U), Tavon_Calc/4(iPhase_U)
  iPhase_V/1 -> DeltaTimeOnOffDuty_Calc/2(iPhase_V), Tavon_Calc/5(iPhase_V)
  iPhase_W/1 -> DeltaTimeOnOffDuty_Calc/3(iPhase_W), Tavon_Calc/6(iPhase_W)
  uDcLink/1 -> Tavon_Calc/7(uDcLink)
  PwmFreq_Hz/1 -> DeadTimeDuty_Calc/1(PwmFreq_Hz), DeltaTimeOnOffDuty_Calc/4(PwmFreq_Hz)
  Tavon_Calc/1(Bus_DutyAvon) -> Bus Creator/2  "Bus_DutyAvon"
  DeltaTimeOnOffDuty_Calc/1(Bus_DeltaTimeOnOffDuty) -> Bus Creator/3  "Bus_DeltaTimeOnOffDuty"
  DeadTimeDuty_Calc/1(DeadTimeDuty_NULL) -> Bus Creator/4  "DeadTimeDuty_NULL"
  Bus Creator/1 -> Bus_DutyCompensate/1  "Bus_DutyCompensate"
  Bus Creator1/1 -> Bus Creator/1  "SVM_DutyPhase"

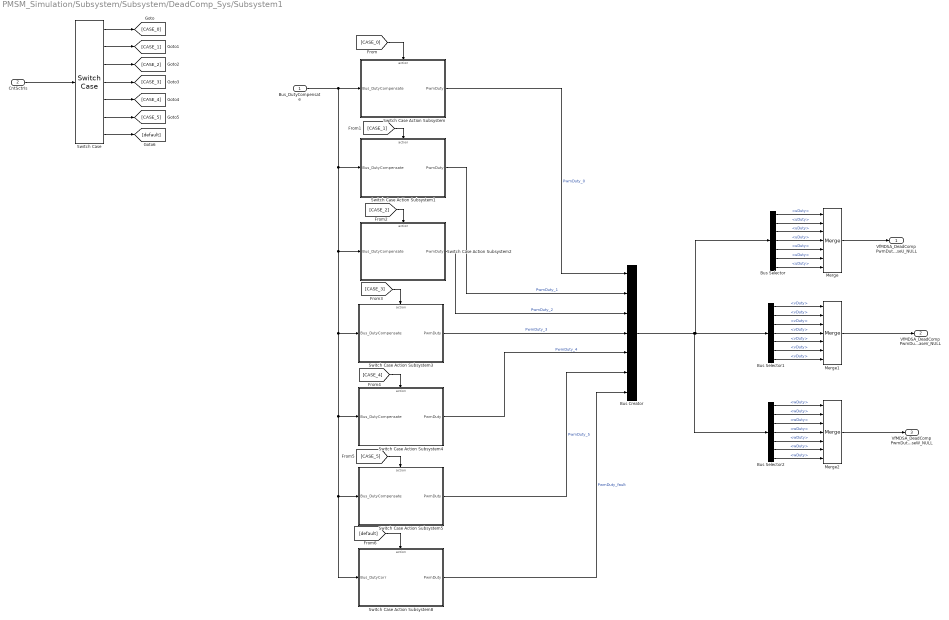
== system PMSM_Simulation/Subsystem/Subsystem/DeadComp_Sys/Subsystem1 ==
  Bus_DutyCompensate : Inport
  CntSctrIs : Inport  Port=2
  Bus Creator : BusCreator  Inputs=7
  Bus Selector : BusSelector  OutputSignals=PwmDuty_0.uDuty,PwmDuty_1.uDuty,PwmDuty_2.uDuty,PwmDuty_3.uDuty,PwmDuty_4.uDuty,PwmDuty_5.uDuty,PwmDuty_fault.uDuty
  Bus Selector1 : BusSelector  OutputSignals=PwmDuty_1.vDuty,PwmDuty_0.vDuty,PwmDuty_2.vDuty,PwmDuty_3.vDuty,PwmDuty_4.vDuty,PwmDuty_5.vDuty,PwmDuty_fault.vDuty
  Bus Selector2 : BusSelector  OutputSignals=PwmDuty_0.wDuty,PwmDuty_1.wDuty,PwmDuty_2.wDuty,PwmDuty_3.wDuty,PwmDuty_4.wDuty,PwmDuty_5.wDuty,PwmDuty_fault.wDuty
  Merge : Merge  Inputs=7
  Merge1 : Merge  Inputs=7
  Merge2 : Merge  Inputs=7
  Switch Case : SwitchCase  CaseConditions={0,1,2,3,4,5}
  Switch Case Action Subsystem : Subsystem  TreatAsAtomicUnit=on
  Switch Case Action Subsystem1 : Subsystem  TreatAsAtomicUnit=on
  Switch Case Action Subsystem2 : Subsystem  TreatAsAtomicUnit=on
  Switch Case Action Subsystem3 : Subsystem  TreatAsAtomicUnit=on
  Switch Case Action Subsystem4 : Subsystem  TreatAsAtomicUnit=on
  Switch Case Action Subsystem5 : Subsystem  TreatAsAtomicUnit=on
  Switch Case Action Subsystem8 : Subsystem  TreatAsAtomicUnit=on
  VfMDSA_DeadCompPwmDutyCyclePhaseU_NULL : Outport
  VfMDSA_DeadCompPwmDutyCyclePhaseV_NULL : Outport  Port=2
  VfMDSA_DeadCompPwmDutyCyclePhaseW_NULL : Outport  Port=3
  wires:
  CntSctrIs/1 -> Switch Case/1
  Switch Case/1 -> [CASE_0]
  Switch Case/2 -> [CASE_1]
  Switch Case/3 -> [CASE_2]
  Switch Case/4 -> [CASE_3]
  Switch Case/5 -> [CASE_4]
  Switch Case/7 -> [default]
  [CASE_0] -> Switch Case Action Subsystem/Action
  [CASE_1] -> Switch Case Action Subsystem1/Action
  [CASE_2] -> Switch Case Action Subsystem2/Action
  [CASE_3] -> Switch Case Action Subsystem3/Action
  [CASE_4] -> Switch Case Action Subsystem4/Action
  [CASE_5] -> Switch Case Action Subsystem5/Action
  [default] -> Switch Case Action Subsystem8/Action
  Switch Case/6 -> [CASE_5]
  Merge/1 -> VfMDSA_DeadCompPwmDutyCyclePhaseU_NULL/1
  Switch Case Action Subsystem/1(PwmDuty) -> Bus Creator/1  "PwmDuty_0"
  Switch Case Action Subsystem1/1(PwmDuty) -> Bus Creator/2  "PwmDuty_1"
  Switch Case Action Subsystem2/1(PwmDuty) -> Bus Creator/3  "PwmDuty_2"
  Switch Case Action Subsystem3/1(PwmDuty) -> Bus Creator/4  "PwmDuty_3"
  Switch Case Action Subsystem4/1(PwmDuty) -> Bus Creator/5  "PwmDuty_4"
  Switch Case Action Subsystem5/1(PwmDuty) -> Bus Creator/6  "PwmDuty_5"
  Switch Case Action Subsystem8/1(PwmDuty) -> Bus Creator/7  "PwmDuty_fault"
  Merge1/1 -> VfMDSA_DeadCompPwmDutyCyclePhaseV_NULL/1
  Merge2/1 -> VfMDSA_DeadCompPwmDutyCyclePhaseW_NULL/1
  Bus Creator/1 -> Bus Selector2/1, Bus Selector1/1, Bus Selector/1
  Bus Selector/1 -> Merge/1  "<uDuty>"
  Bus Selector/2 -> Merge/2  "<uDuty>"
  Bus Selector/3 -> Merge/3  "<uDuty>"
  Bus Selector/4 -> Merge/4  "<uDuty>"
  Bus Selector/5 -> Merge/5  "<uDuty>"
  Bus Selector/6 -> Merge/6  "<uDuty>"
  Bus Selector/7 -> Merge/7  "<uDuty>"
  Bus Selector1/1 -> Merge1/1  "<vDuty>"
  Bus Selector1/2 -> Merge1/2  "<vDuty>"
  Bus Selector1/3 -> Merge1/3  "<vDuty>"
  Bus Selector1/4 -> Merge1/4  "<vDuty>"
  Bus Selector1/5 -> Merge1/5  "<vDuty>"
  Bus Selector1/6 -> Merge1/6  "<vDuty>"
  Bus Selector1/7 -> Merge1/7  "<vDuty>"
  Bus Selector2/1 -> Merge2/1  "<wDuty>"
  Bus Selector2/2 -> Merge2/2  "<wDuty>"
  Bus Selector2/3 -> Merge2/3  "<wDuty>"
  Bus Selector2/4 -> Merge2/4  "<wDuty>"
  Bus Selector2/5 -> Merge2/5  "<wDuty>"
  Bus Selector2/6 -> Merge2/6  "<wDuty>"
  Bus Selector2/7 -> Merge2/7  "<wDuty>"
  Bus_DutyCompensate/1 -> Switch Case Action Subsystem1/1(Bus_DutyCompensate), Switch Case Action Subsystem2/1(Bus_DutyCompensate), Switch Case Action Subsystem3/1(Bus_DutyCompensate), Switch Case Action Subsystem4/1(Bus_DutyCompensate), Switch Case Action Subsystem5/1(Bus_DutyCompensate), Switch Case Action Subsystem8/1("Bus_DutyCorr "), Switch Case Action Subsystem/1(Bus_DutyCompensate)

== system PMSM_Simulation/Subsystem/Subsystem/DeadComp_Sys/Subsystem2 ==
  IsdDes_A : Inport
  IsqDes_A : Inport  Port=2
  IsdFb_A : Inport  Port=3
  IsqFb_A : Inport  Port=4
  FrqRtrEl_Hz : Inport  Port=5
  agPreRtrEl : Inport  Port=6
  PwmFreq_Hz : Inport  Port=7
  Gain : Gain  Gain=6*pi
  Inverse Clarke Transform : mcbcontrolslib/Inverse Clarke Transform
  Inverse Park Transform : mcbcontrolslib/Inverse Park Transform  AxisAlignment=D-axis
  Sine-Cosine Lookup : mcbcontrolslib/Sine-Cosine Lookup  AngleInput=Radians  N_points=4095
  Subsystem1 : Subsystem
  Subsystem3 : Subsystem
  iaPre : Outport
  ibPre : Outport  Port=2
  icPre : Outport  Port=3
  CntSctrIs : Outport  Port=4
  wires:
  Inverse Park Transform/1 -> Inverse Clarke Transform/1
  Subsystem1/2(Isq_A) -> Inverse Park Transform/2, Subsystem3/5(Isq_A)
  IsdDes_A/1 -> Subsystem1/1(IsdDes_A)
  Subsystem1/1(Isd_A) -> Inverse Park Transform/1, Subsystem3/4(Isd_A)
  Sine-Cosine Lookup/2 -> Inverse Park Transform/4
  Inverse Clarke Transform/2 -> ibPre/1
  Sine-Cosine Lookup/1 -> Inverse Park Transform/3
  IsqFb_A/1 -> Subsystem1/4(IsqFb_A)
  Inverse Clarke Transform/3 -> icPre/1
  Inverse Park Transform/2 -> Inverse Clarke Transform/2
  IsdFb_A/1 -> Subsystem1/3(IsdFb_A)
  FrqRtrEl_Hz/1 -> Gain/1
  IsqDes_A/1 -> Subsystem1/2(IsqDes_A)
  agPreRtrEl/1 -> Subsystem3/2(eMtrPos_NULL)
  Inverse Clarke Transform/1 -> iaPre/1
  PwmFreq_Hz/1 -> Subsystem3/3(VfPwmFreq_Hz)
  Gain/1 -> Subsystem3/1(eMtrSpd_rads)
  Subsystem3/2(Select_N) -> CntSctrIs/1
  Subsystem3/1(PreMtrPos) -> Sine-Cosine Lookup/1

== system PMSM_Simulation/Subsystem/Subsystem/SMO/Subsystem ==
  Ualpha : Inport
  iAlpha : Inport  Port=2
  we : Inport  Port=3
  iBeta‘ : Inport  Port=4
  Add : Sum  Inputs=+---
  Discrete-Time Integrator : DiscreteIntegrator  SampleTime=-1  ICPrevOutput=DiscIntNeverNeededParam  ICPrevScaledInput=DiscIntNeverNeededParam
  Gain : Gain  Gain=1/Ld
  Gain1 : Gain  Gain=Rs/Ld
  Gain2 : Gain  Gain=SMO_Kp
  Gain3 : Gain  Gain=(Ld-Lq)/Ld
  Gain4 : Gain  Gain=1/Ld
  IIR Filter : mcbcontrolslib/IIR Filter  VariantControl=Low Pass Filter  VariantSelect=Low-pass  Filter_constant=0.0001  advancedSettings=off  Ts=50e-6  cutOff_freq=0.31834
      settings: LibrarySourceBlock=mcbhdllib/Signal Management/IIR Filter
  Product : Product
  Sign : Signum
  Subsystem : Subsystem
  Sum : Sum  Inputs=|+-
  Ealpha : Outport
  Ialpha’ : Outport  Port=2
  wires:
  Ualpha/1 -> Gain/1
  Gain/1 -> Add/1
  Gain1/1 -> Add/3
  Add/1 -> Discrete-Time Integrator/1
  Sum/1 -> Sign/1
  Discrete-Time Integrator/1 -> Gain1/1, Sum/1, Ialpha’/1  "Ialpha’"
  iAlpha/1 -> Sum/2
  Gain2/1 -> Subsystem/1(In1), IIR Filter/1, Gain4/1
  Sign/1 -> Gain2/1
  we/1 -> Product/1
  iBeta‘/1 -> Product/2
  Product/1 -> Gain3/1
  Gain3/1 -> Add/2
  Gain4/1 -> Add/4
  Subsystem/1(Ealpha) -> Ealpha/1

== system PMSM_Simulation/Subsystem/Subsystem/SMO/Subsystem1 ==
  iAlpha' : Inport
  we : Inport  Port=2
  Ubeta : Inport  Port=3
  iBeta : Inport  Port=4
  Add : Sum  Inputs=++--
  Discrete-Time Integrator : DiscreteIntegrator  SampleTime=-1  ICPrevOutput=DiscIntNeverNeededParam  ICPrevScaledInput=DiscIntNeverNeededParam
  Gain : Gain  Gain=1/Lq
  Gain1 : Gain  Gain=Rs/Lq
  Gain2 : Gain  Gain=SMO_Kp
  Gain3 : Gain  Gain=(Ld-Lq)/Lq
  Gain4 : Gain  Gain=1/Lq
  Product : Product
  Sign : Signum
  Subsystem : Subsystem
  Sum : Sum  Inputs=|+-
  iBeta’ : Outport
  Ebeta : Outport  Port=2
  wires:
  Product/1 -> Gain3/1
  Gain1/1 -> Add/3
  Sum/1 -> Sign/1
  Gain3/1 -> Add/2
  Add/1 -> Discrete-Time Integrator/1
  Sign/1 -> Gain2/1
  Gain2/1 -> Subsystem/1(In1), Gain4/1
  iBeta/1 -> Sum/2
  Gain/1 -> Add/1
  Ubeta/1 -> Gain/1
  Discrete-Time Integrator/1 -> Gain1/1, iBeta’/1, Sum/1  "iBeta'"
  we/1 -> Product/1
  iAlpha'/1 -> Product/2
  Gain4/1 -> Add/4
  Subsystem/1(Ealpha) -> Ebeta/1

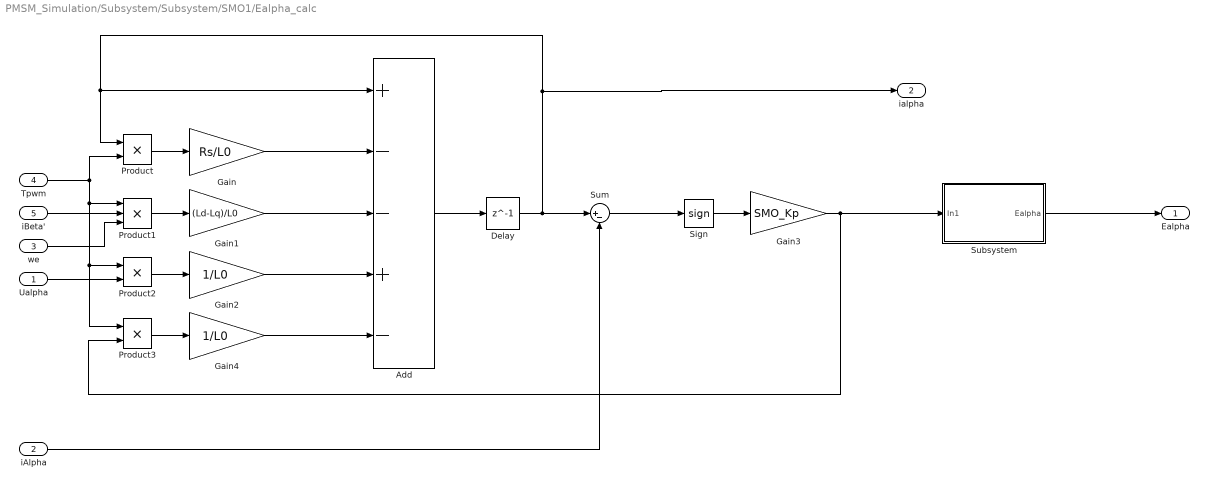
== system PMSM_Simulation/Subsystem/Subsystem/SMO1/Ealpha_calc ==
  Ualpha : Inport
  iAlpha : Inport  Port=2
  we : Inport  Port=3
  Tpwm : Inport  Port=4
  iBeta' : Inport  Port=5
  Add : Sum  Inputs=+--+-
  Delay : Delay  DelayLength=1
  Gain : Gain  Gain=Rs/L0
  Gain1 : Gain  Gain=(Ld-Lq)/L0
  Gain2 : Gain  Gain=1/L0
  Gain3 : Gain  Gain=SMO_Kp
  Gain4 : Gain  Gain=1/L0
  Product : Product
  Product1 : Product  Inputs=3
  Product2 : Product
  Product3 : Product
  Sign : Signum
  Subsystem : Subsystem
  Sum : Sum  Inputs=|+-
  Ealpha : Outport
  ialpha : Outport  Port=2
  wires:
  Add/1 -> Delay/1
  Delay/1 -> Sum/1, ialpha/1, Product/1, Add/1
  Product/1 -> Gain/1
  Tpwm/1 -> Product/2, Product1/1, Product3/1, Product2/1
  Gain/1 -> Add/2
  iBeta'/1 -> Product1/2
  Product1/1 -> Gain1/1
  Gain1/1 -> Add/3
  we/1 -> Product1/3
  Ualpha/1 -> Product2/2
  Product2/1 -> Gain2/1
  Gain2/1 -> Add/4
  Sign/1 -> Gain3/1
  Gain3/1 -> Product3/2, Subsystem/1(In1)
  Sum/1 -> Sign/1
  iAlpha/1 -> Sum/2
  Gain4/1 -> Add/5
  Product3/1 -> Gain4/1
  Subsystem/1(Ealpha) -> Ealpha/1

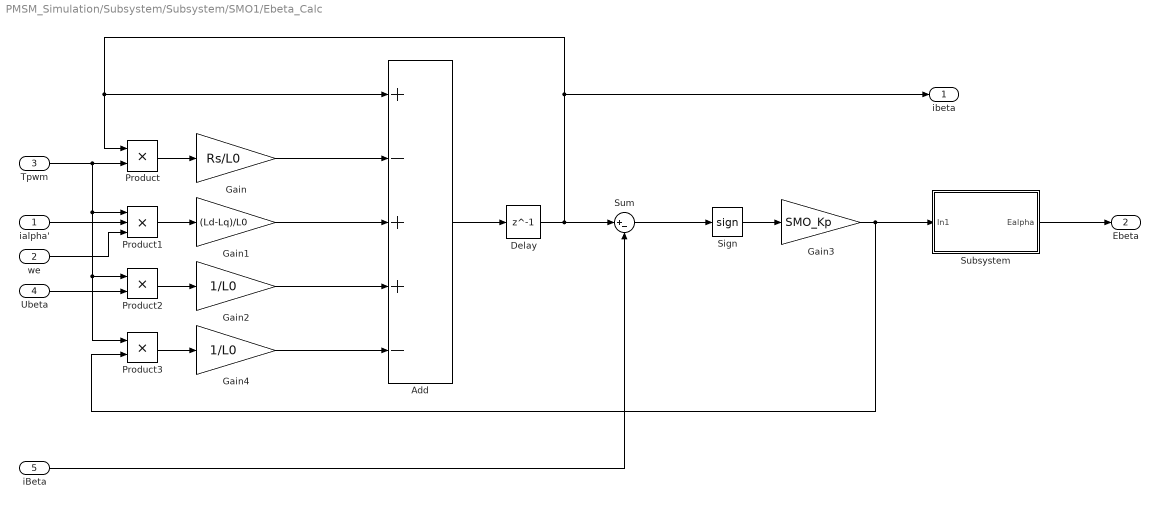
== system PMSM_Simulation/Subsystem/Subsystem/SMO1/Ebeta_Calc ==
  ialpha' : Inport
  we : Inport  Port=2
  Tpwm : Inport  Port=3
  Ubeta : Inport  Port=4
  iBeta : Inport  Port=5
  Add : Sum  Inputs=+-++-
  Delay : Delay  DelayLength=1
  Gain : Gain  Gain=Rs/L0
  Gain1 : Gain  Gain=(Ld-Lq)/L0
  Gain2 : Gain  Gain=1/L0
  Gain3 : Gain  Gain=SMO_Kp
  Gain4 : Gain  Gain=1/L0
  Product : Product
  Product1 : Product  Inputs=3
  Product2 : Product
  Product3 : Product
  Sign : Signum
  Subsystem : Subsystem
  Sum : Sum  Inputs=|+-
  ibeta : Outport
  Ebeta : Outport  Port=2
  wires:
  Delay/1 -> Sum/1, ibeta/1, Product/1, Add/1
  Product3/1 -> Gain4/1
  Gain1/1 -> Add/3
  Product/1 -> Gain/1
  Ubeta/1 -> Product2/2
  Gain/1 -> Add/2
  Gain3/1 -> Subsystem/1(In1), Product3/2
  ialpha'/1 -> Product1/2
  Gain2/1 -> Add/4
  Tpwm/1 -> Product1/1, Product3/1, Product2/1, Product/2
  iBeta/1 -> Sum/2
  Product1/1 -> Gain1/1
  Sum/1 -> Sign/1
  Add/1 -> Delay/1
  Product2/1 -> Gain2/1
  Sign/1 -> Gain3/1
  we/1 -> Product1/3
  Gain4/1 -> Add/5
  Subsystem/1(Ealpha) -> Ebeta/1

== system PMSM_Simulation/Subsystem/Subsystem/SVM_PU/N_Sector_calc ==
  Ualpha : Inport
  Ubeta : Inport  Port=2
  N_calc : Subsystem
  Uref_Calc : Subsystem
  N_Sector : Outport
  wires:
  Uref_Calc/2(Uref2) -> N_calc/2(Uref2)
  Ualpha/1 -> Uref_Calc/1(Ualpha)
  Ubeta/1 -> Uref_Calc/2(Ubeta)
  Uref_Calc/3(Uref3) -> N_calc/3(Uref3)
  N_calc/1(N_Sector) -> N_Sector/1
  Uref_Calc/1(Uref1) -> N_calc/1(Uref1)

== system PMSM_Simulation/Subsystem/Subsystem/SVM_PU/Subsystem ==
  Ualpha : Inport
  Ubeta : Inport  Port=2
  Add1 : Sum
  Add2 : Sum  Inputs=-+
  ConstanT1 : Constant  Value=2  OutDataTypeStr=single
  ConstanT2 : Constant  Value=sqrt(3)/2  OutDataTypeStr=single
  Constant : Constant  Value=3/2  OutDataTypeStr=single
  ProducT1 : Product
  ProducT2 : Product
  Product : Product
  X : Outport
  Y : Outport  Port=2
  Z : Outport  Port=3
  wires:
  Ualpha/1 -> Product/1
  Constant/1 -> Product/2
  ProducT1/1 -> X/1
  ConstanT1/1 -> ProducT1/2
  Ubeta/1 -> ProducT2/1
  Add1/1 -> Y/1
  Product/1 -> Add2/1, Add1/1
  ProducT2/1 -> ProducT1/1, Add2/2, Add1/2
  ConstanT2/1 -> ProducT2/2
  Add2/1 -> Z/1

== system PMSM_Simulation/Subsystem/Subsystem/SVM_PU/Subsystem1 ==
  T1 : Inport
  T2 : Inport  Port=2
  Add : Sum  Inputs=+--
  Add1 : Sum  Inputs=++-
  Add2 : Sum  Inputs=+++
  Constant : Constant  Value=1/4  OutDataTypeStr=single
  Gain1 : Gain  Gain=1/4
  Gain2 : Gain  Gain=1/4
  Ta : Outport
  Tb : Outport  Port=2
  Tc : Outport  Port=3
  wires:
  T1/1 -> Gain1/1
  T2/1 -> Gain2/1
  Constant/1 -> Add2/1, Add1/1, Add/1
  Add/1 -> Ta/1
  Gain1/1 -> Add2/2, Add1/2, Add/2
  Gain2/1 -> Add1/3, Add2/3, Add/3
  Add1/1 -> Tb/1
  Add2/1 -> Tc/1

== system PMSM_Simulation/Subsystem/Subsystem/SVM_PU/T1_T2_Calc ==
  N_Sector : Inport
  X : Inport  Port=2
  Y : Inport  Port=3
  Z : Inport  Port=4
  Subsystem1 : Subsystem
  Subsystem2 : Subsystem
  T4_T6 : Subsystem  Commented=on
  T1 : Outport
  T2 : Outport  Port=2
  wires:
  X/1 -> Subsystem1/2(X)
  Z/1 -> Subsystem1/4(Z)
  N_Sector/1 -> Subsystem1/1(N_Sector)
  Y/1 -> Subsystem1/3(Y)
  Subsystem1/1(Bus_T4T6) -> Subsystem2/1(Bus_T4T6)
  Subsystem2/1(T1) -> T1/1
  Subsystem2/2(T2) -> T2/1

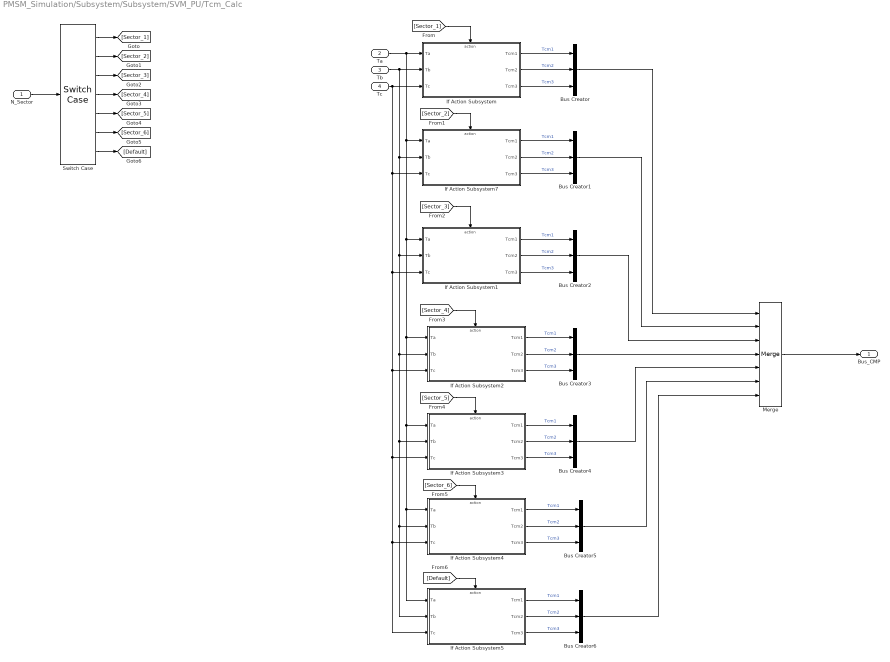
== system PMSM_Simulation/Subsystem/Subsystem/SVM_PU/Tcm_Calc ==
  N_Sector : Inport
  Ta : Inport  Port=2
  Tb : Inport  Port=3
  Tc : Inport  Port=4
  Bus Creator{,1..6} (7 alike) : BusCreator  Inputs=3
  If Action Subsystem : Subsystem  TreatAsAtomicUnit=on
  If Action Subsystem1 : Subsystem  TreatAsAtomicUnit=on
  If Action Subsystem2 : Subsystem  TreatAsAtomicUnit=on
  If Action Subsystem3 : Subsystem  TreatAsAtomicUnit=on
  If Action Subsystem4 : Subsystem  TreatAsAtomicUnit=on
  If Action Subsystem5 : Subsystem  TreatAsAtomicUnit=on
  If Action Subsystem7 : Subsystem  TreatAsAtomicUnit=on
  Merge : Merge  Inputs=7
  Switch Case : SwitchCase  CaseConditions={1,2,3,4,5,6}
  Bus_CMP : Outport
  wires:
  Switch Case/1 -> [Sector_1]
  Switch Case/2 -> [Sector_2]
  Switch Case/4 -> [Sector_4]
  Switch Case/6 -> [Sector_6]
  Switch Case/3 -> [Sector_3]
  N_Sector/1 -> Switch Case/1
  Switch Case/7 -> [Default]
  Switch Case/5 -> [Sector_5]
  [Sector_1] -> If Action Subsystem/Action
  [Sector_2] -> If Action Subsystem7/Action
  [Sector_4] -> If Action Subsystem2/Action
  [Sector_3] -> If Action Subsystem1/Action
  [Sector_6] -> If Action Subsystem4/Action
  [Sector_5] -> If Action Subsystem3/Action
  [Default] -> If Action Subsystem5/Action
  Tb/1 -> If Action Subsystem5/2(Tb), If Action Subsystem4/2(Tb), If Action Subsystem3/2(Tb), If Action Subsystem2/2(Tb), If Action Subsystem1/2(Tb), If Action Subsystem7/2(Tb), If Action Subsystem/2(Tb)
  Tc/1 -> If Action Subsystem/3(Tc), If Action Subsystem5/3(Tc), If Action Subsystem4/3(Tc), If Action Subsystem3/3(Tc), If Action Subsystem2/3(Tc), If Action Subsystem1/3(Tc), If Action Subsystem7/3(Tc)
  Ta/1 -> If Action Subsystem5/1(Ta), If Action Subsystem4/1(Ta), If Action Subsystem3/1(Ta), If Action Subsystem2/1(Ta), If Action Subsystem1/1(Ta), If Action Subsystem7/1(Ta), If Action Subsystem/1(Ta)
  Merge/1 -> Bus_CMP/1
  If Action Subsystem/1(Tcm1) -> Bus Creator/1  "Tcm1"
  If Action Subsystem/2(Tcm2) -> Bus Creator/2  "Tcm2"
  If Action Subsystem/3(Tcm3) -> Bus Creator/3  "Tcm3"
  If Action Subsystem7/1(Tcm1) -> Bus Creator1/1  "Tcm1"
  If Action Subsystem7/3(Tcm3) -> Bus Creator1/3  "Tcm3"
  If Action Subsystem7/2(Tcm2) -> Bus Creator1/2  "Tcm2"
  If Action Subsystem1/1(Tcm1) -> Bus Creator2/1  "Tcm1"
  If Action Subsystem1/3(Tcm3) -> Bus Creator2/3  "Tcm3"
  If Action Subsystem1/2(Tcm2) -> Bus Creator2/2  "Tcm2"
  If Action Subsystem2/1(Tcm1) -> Bus Creator3/1  "Tcm1"
  If Action Subsystem2/3(Tcm3) -> Bus Creator3/3  "Tcm3"
  If Action Subsystem2/2(Tcm2) -> Bus Creator3/2  "Tcm2"
  If Action Subsystem3/1(Tcm1) -> Bus Creator4/1  "Tcm1"
  If Action Subsystem3/3(Tcm3) -> Bus Creator4/3  "Tcm3"
  If Action Subsystem3/2(Tcm2) -> Bus Creator4/2  "Tcm2"
  If Action Subsystem4/1(Tcm1) -> Bus Creator5/1  "Tcm1"
  If Action Subsystem4/3(Tcm3) -> Bus Creator5/3  "Tcm3"
  If Action Subsystem4/2(Tcm2) -> Bus Creator5/2  "Tcm2"
  If Action Subsystem5/1(Tcm1) -> Bus Creator6/1  "Tcm1"
  If Action Subsystem5/3(Tcm3) -> Bus Creator6/3  "Tcm3"
  If Action Subsystem5/2(Tcm2) -> Bus Creator6/2  "Tcm2"
  Bus Creator/1 -> Merge/1
  Bus Creator1/1 -> Merge/2
  Bus Creator2/1 -> Merge/3
  Bus Creator3/1 -> Merge/4
  Bus Creator4/1 -> Merge/5
  Bus Creator5/1 -> Merge/6
  Bus Creator6/1 -> Merge/7
